simulink model "nonlinear_closed_observer_redused"  (R2024a)
settings: Solver=VariableStepAuto  StartTime=0.0  StopTime=15.0  MaxStep=1e-3  RelTol=1e-3
values from neighbouring files (symbols this model uses):
  B = [0; J / ((M+m)*J - beta^2); 0; -beta / ((M+m)*J - beta^2)]    [nonlinear_with_observer.m]    (also in nonlinear_with_reduced_observer.m = [0; J/Delta0; 0; -beta/Delta0]; t_31.m = [0; J/Meff; 0; -beta/Meff]; t_311.m = [0; J/Meff; 0; -beta/Meff]; t_312.m = [0; J/Meff; 0; -beta/Meff])
  beta = m * lc    (= 40.0551)    [t_31.m]    (also in t_311.m; t_312.m; t_32.m; t_321.m)
  f = 0    [nonlinear_model_closed.m]    (also in nonlinear_with_observer.m; nonlinear_with_reduced_observer.m; t_312.m; t_32.m)
  g = 9.81    [t_31.m]    (also in t_311.m; t_312.m; t_32.m; t_321.m)
  Gamma = diag(lam_red)    [design_reduced_observer.m]    (also in t_32.m = diag(lam_obs))
  J = (1/3)*m1*l^2 + m2*l^2    (= 62.720658)    [t_31.m]    (also in t_311.m; t_312.m; t_32.m; t_321.m)
  K = [0 0 0 1] * inv(U) * D_A    [t_31.m]    (also in t_311.m = 1.0e+04*[-0.0046   -0.0233   -1.0984   -0.3688]; t_312.m = acker(A, B, lamJe); t_32.m = [-46.28, -233.21, -10984.45, -3688.10]; t_321.m = [-46.28, -233.21, -10984.45, -3688.10])
  M = 658.36    [t_31.m]    (also in t_311.m; t_312.m; t_32.m; t_321.m)
  m = m1 + m2    (= 30.46)    [t_31.m]    (also in t_311.m; t_312.m; t_32.m; t_321.m)
  Q = double([sol.q11, 1, sol.q12, 0 ... (first row only)    [design_reduced_observer.m]    (also in t_32.m = [q11, 1, q13, 0)
  T_inv = inv(T)    [design_reduced_observer.m]    (also in t_32.m)
  x0 = x0_list{i}    [t_31.m]    (also in t_311.m; t_312.m = [0.1; 0.2; 0.03; 0.12]; t_32.m = [0.1; 0.2; 0.03; 0.12]; t_321.m = [0.1; 0.2; 0.03; 0.12])
  Y = (Gamma * Q - Q * A) * pinv(C)    [design_reduced_observer.m]    (also in t_32.m)
  z0 = [x0; x_hat0]    [design_full_observer.m]    (also in design_reduced_observer.m = [x0; z_hat0]; t_32.m = [-0; -0])
settings Model: Creator=eva  LastModifiedBy=eva

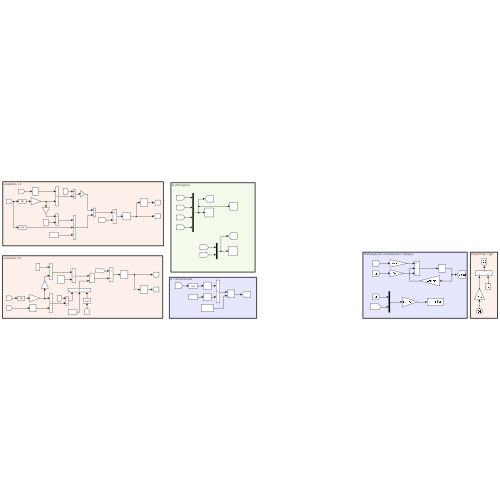
[thumbnail: Simulink's stored preview of the top-level diagram]
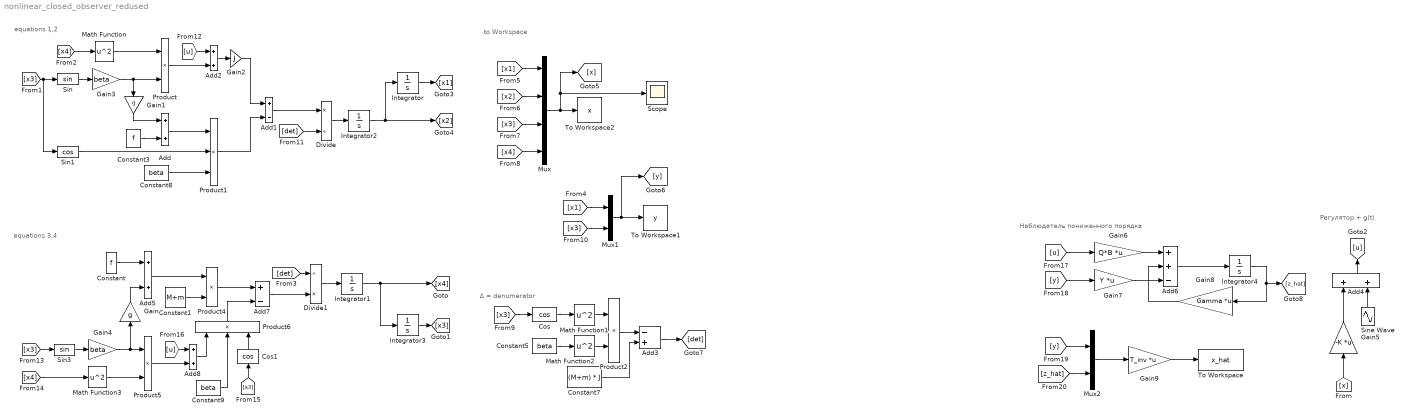
== system nonlinear_closed_observer_redused ==
  note: Регулятор + g(t)
  note: equations 3,4
  note: to Workspace
  note: Наблюдатель пониженного порядка
  note: Δ = denumerator
  note: equations 1,2
  Add{,2,4..5,8} (5 alike) : Sum
  Add1 : Sum  Inputs=+-
  Add3 : Sum  Inputs=-+
  Add6 : Sum  Inputs=++-
  Add7 : Sum  Inputs=+-
  Constant : Constant  Value=f
  Constant1 : Constant  Value=M+m
  Constant3 : Constant  Value=f
  Constant5 : Constant  Value=beta
  Constant7 : Constant  Value=(M+m) * J
  Constant8 : Constant  Value=beta
  Constant9 : Constant  Value=beta
  Cos : Trigonometry  Operator=cos
  Cos1 : Trigonometry  Operator=cos
  Divide : Product  Inputs=*/
  Divide1 : Product  Inputs=/*
  Gain : Gain  Gain=g
  Gain1 : Gain  Gain=g
  Gain2 : Gain  Gain=J
  Gain3 : Gain  Gain=beta
  Gain4 : Gain  Gain=beta
  Gain5 : Gain  Gain=-K  Multiplication=Matrix(K*u)
  Gain6 : Gain  Gain=Q*B  Multiplication=Matrix(K*u)
  Gain7 : Gain  Gain=Y  Multiplication=Matrix(K*u)
  Gain8 : Gain  Gain=Gamma  Multiplication=Matrix(K*u)
  Gain9 : Gain  Gain=T_inv  Multiplication=Matrix(K*u)
  Integrator : Integrator  InitialCondition=x0(1)
  Integrator1 : Integrator  InitialCondition=x0(4)
  Integrator2 : Integrator  InitialCondition=x0(2)
  Integrator3 : Integrator  InitialCondition=x0(3)
  Integrator4 : Integrator  InitialCondition=z0
  Math Function{,1..3} (4 alike) : Math  Operator=square
  Mux : Mux
  Mux1 : Mux  Inputs=2
  Mux2 : Mux  Inputs=2
  Product{,2,4..5} (4 alike) : Product
  Product1 : Product  Inputs=3
  Product6 : Product  Inputs=3
  Scope : Scope
  Sin : Trigonometry
  Sin1 : Trigonometry  Operator=cos
  Sin3 : Trigonometry
  Sine Wave : Sin  Amplitude=0  Frequency=0  SampleTime=0
  To Workspace : ToWorkspace  VariableName=x_hat  SaveFormat=Structure With Time  SampleTime=-1
  To Workspace1 : ToWorkspace  VariableName=y  SaveFormat=Structure With Time  SampleTime=-1
  To Workspace2 : ToWorkspace  VariableName=x  SaveFormat=Structure With Time  SampleTime=-1
  wires:
  Gain1/1 -> Add/1
  Integrator2/1 -> [x2], Integrator/1
  Constant5/1 -> Math Function2/1
  Integrator3/1 -> [x3]
  [x3] -> Sin3/1
  [x3] -> Mux1/2
  Divide/1 -> Integrator2/1
  Math Function2/1 -> Product2/2
  Product6/1 -> Add7/2
  [x4] -> Math Function/1
  Math Function/1 -> Product/1
  [x1] -> Mux1/1
  [u] -> Add8/1
  Constant8/1 -> Product1/3
  [det] -> Divide/2
  Add2/1 -> Gain2/1
  [x3] -> Sin/1, Sin1/1
  Gain4/1 -> Product5/1, Gain/1
  Sin/1 -> Gain3/1
  Sine Wave/1 -> Add4/2
  Add5/1 -> Product4/1
  Math Function3/1 -> Product5/2
  Product2/1 -> Add3/1
  [det] -> Divide1/1
  Gain5/1 -> Add4/1
  Divide1/1 -> Integrator1/1
  Add3/1 -> [det]
  Add/1 -> Product1/1
  [u] -> Add2/1
  Gain2/1 -> Add1/1
  Sin1/1 -> Product1/2
  [x3] -> Cos/1
  Product4/1 -> Add7/1
  Gain3/1 -> Product/2, Gain1/1
  Add8/1 -> Product6/1
  Product/1 -> Add2/2
  Constant7/1 -> Add3/2
  Mux1/1 -> [y], To Workspace1/1
  Sin3/1 -> Gain4/1
  Add4/1 -> [u]
  Add1/1 -> Divide/1
  Cos/1 -> Math Function1/1
  Integrator1/1 -> [x4], Integrator3/1
  Integrator/1 -> [x1]
  [x2] -> Mux/2
  [x] -> Gain5/1
  Product5/1 -> Add8/2
  [x3] -> Mux/3
  [x1] -> Mux/1
  Cos1/1 -> Product6/3
  Add7/1 -> Divide1/2
  [x4] -> Mux/4
  [x4] -> Math Function3/1
  Math Function1/1 -> Product2/1
  Constant3/1 -> Add/2
  Constant9/1 -> Product6/2
  Product1/1 -> Add1/2
  Gain/1 -> Add5/2
  Constant/1 -> Add5/1
  [x3] -> Cos1/1
  Mux/1 -> [x], Scope/1, To Workspace2/1
  Constant1/1 -> Product4/2
  [u] -> Gain6/1
  [y] -> Gain7/1
  Gain6/1 -> Add6/1
  Gain7/1 -> Add6/3
  Add6/1 -> Integrator4/1
  Integrator4/1 -> Gain8/1, [z_hat]
  Gain8/1 -> Add6/2
  [y] -> Mux2/1
  [z_hat] -> Mux2/2
  Mux2/1 -> Gain9/1
  Gain9/1 -> To Workspace/1
